simulink model "Comunicacion_serie"  (R2018a)
settings: Solver=VariableStepAuto  StartTime=0.0  StopTime=inf  RelTol=1e-3
undefined symbols (not defined in the file or in its folder): serial
libraries: instrumentlib x3
settings Model: Creator=Federico  LastModifiedBy=Alan
settings CodeAppCC: StateflowObjectComments=on

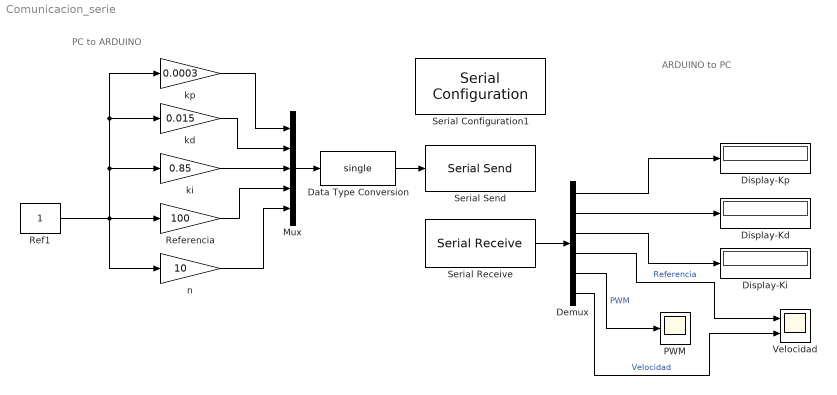
== system Comunicacion_serie ==
  note: PC to ARDUINO
  note: ARDUINO to PC
  Data Type Conversion : DataTypeConversion  OutDataTypeStr=single
  Demux : Demux  Outputs=6
  Display-Kd : Display
  Display-Ki : Display
  Display-Kp : Display
  Mux : Mux  Inputs=5
  PWM : Scope
  Ref1 : Constant  OutDataTypeStr=single  SampleTime=1
  Referencia : Gain  Gain=100
  Serial Configuration1 : instrumentlib/Serial Configuration  Priority=-200000  ComPortMenu=COM3  ComPort=COM3  ObjConstructor=serial('COM3');  BaudRate=115200  DataBits=8  Parity=none  StopBits=1  FlowControl=none  Timeout=10  ByteOrder=LittleEndian
  Serial Receive : instrumentlib/Serial Receive  ComPortMenu=COM3  ComPort=COM3  ObjConstructor=serial('COM3');  Header=efgh  Terminator=<none>  DataSize="[1  6]"  DataType=single  EnableBlockingMode=on  ActionDataUnavailable=Output last received value  CustomValue=0  SampleTime=1
  Serial Send : instrumentlib/Serial Send  ComPortMenu=COM3  ComPort=COM3  ObjConstructor=serial('COM3');  Header=abcd  Terminator=<none>  EnableBlockingMode=on
  Velocidad : Scope  NumInputPorts=2
  kd : Gain  Gain=0.015
  ki : Gain  Gain=0.85
  kp : Gain  Gain=0.0003
  n : Gain  Gain=10
  wires:
  Serial Receive/1 -> Demux/1
  Demux/1 -> Display-Kp/1
  Demux/2 -> Display-Kd/1
  Demux/3 -> Display-Ki/1
  Demux/4 -> Velocidad/1  "Referencia"
  Demux/6 -> Velocidad/2  "Velocidad"
  Demux/5 -> PWM/1  "PWM"
  Data Type Conversion/1 -> Serial Send/1
  Mux/1 -> Data Type Conversion/1
  kp/1 -> Mux/1
  kd/1 -> Mux/2
  ki/1 -> Mux/3
  Referencia/1 -> Mux/4
  n/1 -> Mux/5
  Ref1/1 -> kp/1, kd/1, ki/1, n/1, Referencia/1
